simulink model "EngPrt_TrqLimCalc1"  (R2016b)
settings: configuration reference "CodeGenConfigSet" (kept outside this file)
settings Model: Creator=Administrator  LastModifiedBy=lenovo
settings ConfigSetRef: SourceLocation=Base Workspace

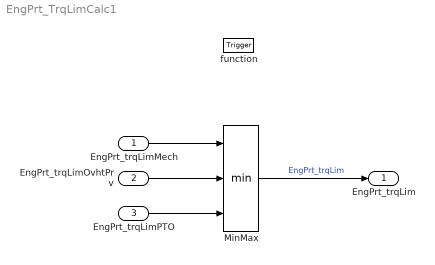
== system EngPrt_TrqLimCalc1 ==
  EngPrt_trqLimMech : Inport  Tag=Nm  Description=Resulting limiting torque for engine mechanics protection (inner engine torque)  OutMin=-3276.8  OutMax=3276.7  OutDataTypeStr=Trq_Nm
  EngPrt_trqLimOvhtPrv : Inport  Tag=Nm  Description=Torque limitation value for engine protection from overheating  Port=2  OutMin=-3276.8  OutMax=3276.7  OutDataTypeStr=Trq_Nm
  EngPrt_trqLimPTO : Inport  Tag=Nm  Description=Torque limitation value from PTO state  Port=3  OutMin=-3276.8  OutMax=3276.7  OutDataTypeStr=Trq_Nm
  function : TriggerPort  TriggerType=function-call  VariantControl=Variant
  MinMax : MinMax  Inputs=3
  EngPrt_trqLim : Outport  Tag=Nm  Description=Limitation torque for engine mechanic protection by torque limitation (as inner engine torque)  OutMin=-3276.8  OutMax=3276.7  OutDataTypeStr=Trq_Nm
  wires:
  MinMax/1 -> EngPrt_trqLim/1  "EngPrt_trqLim"
  EngPrt_trqLimMech/1 -> MinMax/1
  EngPrt_trqLimOvhtPrv/1 -> MinMax/2
  EngPrt_trqLimPTO/1 -> MinMax/3
